simulink model "functions_ex"  (R2020a)
settings: Solver=VariableStepAuto  StartTime=0.0  StopTime=10.0  RelTol=1e-3
settings Model: Creator=lenovo  LastModifiedBy=DELL
settings DataIOCC: ReturnWorkspaceOutputs=off
settings DebuggingCC: ArithmeticOperatorsInVariantConditions=warning
settings SFSimCC: SimUseLocalCustomCode=off  CustomCodeUndefinedFunction=UseInterfaceOnly
settings RTWCC: RTWUseLocalCustomCode=off

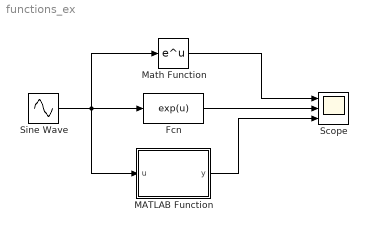
== system functions_ex ==
  Fcn : Fcn  Expr=exp(u)
  MATLAB Function : MATLAB Function  TreatAsAtomicUnit=on
  Math Function : Math  SignedPower=on  SaturateOnIntegerOverflow=on
  Scope : Scope  NumInputPorts=3
  Sine Wave : Sin  SampleTime=0
  wires:
  Sine Wave/1 -> MATLAB Function/1(u), Math Function/1, Fcn/1
  Fcn/1 -> Scope/2
  MATLAB Function/1(y) -> Scope/3
  Math Function/1 -> Scope/1

== matlab function functions_ex/MATLAB Function ==
  data: u input; y output
function y = fcn(u)
y = exp(u);
end
